simulink model "initializeResponseSufrace_th"  (R2018a)
settings: Solver=FixedStepDiscrete  StartTime=0.0  StopTime=10.0  FixedStep=sm.Ts  RelTol=1e-3
libraries: responseSurfaceCharacterization x1
settings Model: Creator=mitch  LastModifiedBy=mitch

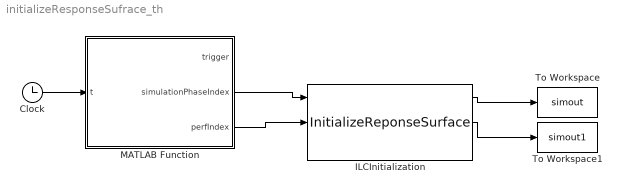
== system initializeResponseSufrace_th ==
  Clock : Clock
  ILCInitialization : responseSurfaceCharacterization/InitializeReponseSurface
  MATLAB Function : MATLAB Function  TreatAsAtomicUnit=on
  To Workspace : ToWorkspace  VariableName=simout  SaveFormat=Timeseries  SampleTime=-1
  To Workspace1 : ToWorkspace  VariableName=simout1  SaveFormat=Timeseries  SampleTime=-1
  wires:
  Clock/1 -> MATLAB Function/1(t)
  MATLAB Function/2(simulationPhaseIndex) -> ILCInitialization/1
  ILCInitialization/1 -> To Workspace/1
  MATLAB Function/3(perfIndex) -> ILCInitialization/2
  ILCInitialization/2 -> To Workspace1/1

== matlab function initializeResponseSufrace_th/MATLAB Function ==
  data: trigger output; t input; simulationPhaseIndex output; perfIndex output
function [trigger, simulationPhaseIndex, perfIndex]  = fcn(t)
persistent count
if isempty(count)
    count = 0;
end
perfIndex = 0;
trigger = false;
if t == 1 || t == 2 || t==3 || t == 4 || t== 5
    trigger = true;
    perfIndex = t;
    count = count+1;
end
simulationPhaseIndex = count;

end
